simulink model "Assembly1"  (R2019b)
settings: Solver=VariableStepAuto  StartTime=0.0  StopTime=100  FixedStep=0.001
model workspace: external: MATLAB File /home/sydney/Desktop/matlab/simulink/SimpImpCheck/Assembly1_DataFile.m (data not in the file)
undefined symbols (not defined in the file or in its folder): smiData, X, Y, Z
libraries: sm_lib x21, fl_lib x17, nesl_utility x17, ee_lib x3
settings Model: Creator=sydney  LastModifiedBy=sydney

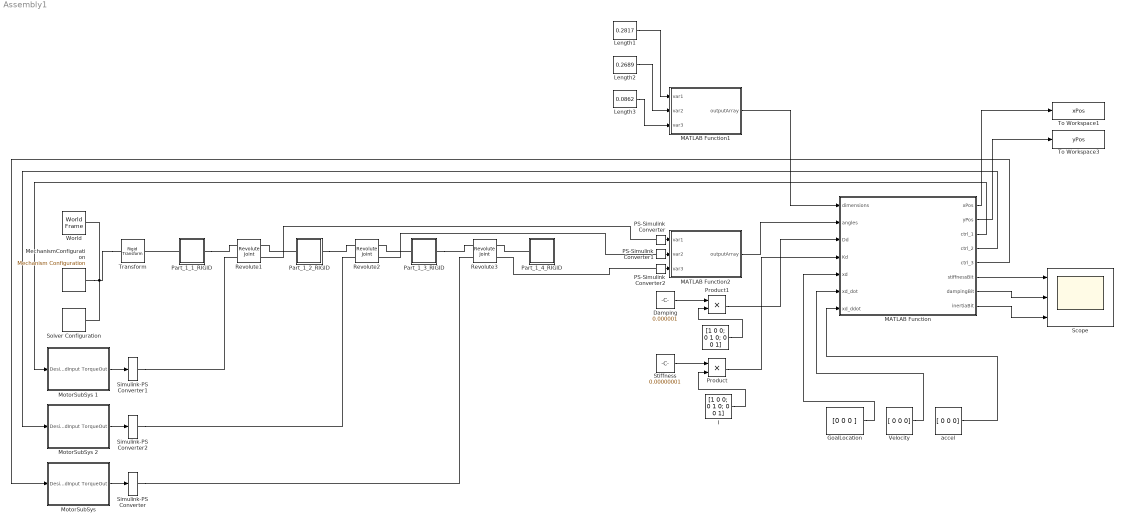
== system Assembly1 ==
  " " : Constant  Value=[1 0 0; 0 1 0; 0 0 1]  VectorParams1D=off
  "Damping " : Constant  Value=0.000001
  GoalLocation : Constant  Value=[0 0 0 ]
  I : Constant  Value=[1 0 0; 0 1 0; 0 0 1]  VectorParams1D=off
  "Length1 " : Constant  Value=0.2817
  "Length2 " : Constant  Value=0.2689
  "Length3 " : Constant  Value=0.0862
  MATLAB Function : MATLAB Function  TreatAsAtomicUnit=on
  MATLAB Function1 : MATLAB Function  TreatAsAtomicUnit=on
  MATLAB Function2 : MATLAB Function  TreatAsAtomicUnit=on
  MechanismConfiguration : sm_lib/Utilities/Mechanism Configuration  UniformGravity=Constant  GravityVector=[0 0 -9.80665]  GravityUnits=m/s^2  LinearizationDelta=0.001
  "MotorSubSys " : Subsystem
  MotorSubSys 1 : Subsystem
  MotorSubSys 2 : Subsystem
  PS-Simulink Converter : nesl_utility/PS-Simulink Converter  PhysicalDomain=network_engine_domain  SubClassName=ps_output  LeftPortType=input  RightPortType=output  PseudoPeriodic=off  Frequencies=[]  Unit=inherit  AffineConversion=off
  PS-Simulink Converter1 : nesl_utility/PS-Simulink Converter  PhysicalDomain=network_engine_domain  SubClassName=ps_output  LeftPortType=input  RightPortType=output  PseudoPeriodic=off  Frequencies=[]  Unit=inherit  AffineConversion=off
  PS-Simulink Converter2 : nesl_utility/PS-Simulink Converter  PhysicalDomain=network_engine_domain  SubClassName=ps_output  LeftPortType=input  RightPortType=output  PseudoPeriodic=off  Frequencies=[]  Unit=inherit  AffineConversion=off
  Part_1_1_RIGID : Subsystem
  Part_1_2_RIGID : Subsystem
  Part_1_3_RIGID : Subsystem
  Part_1_4_RIGID : Subsystem
  Product : Product
  Product1 : Product
  Revolute1 : sm_lib/Joints/Revolute Joint  JointMode=Normal  SenseConstraintForce=off  SenseConstraintForceX=off  SenseConstraintForceY=off  SenseConstraintForceZ=off  SenseConstraintTorque=off  SenseConstraintTorqueX=off  SenseConstraintTorqueY=off  SenseConstraintTorqueZ=off  SenseTotalForce=off  SenseTotalForceX=off  SenseTotalForceY=off  SenseTotalForceZ=off  SenseTotalTorque=off  SenseTotalTorqueX=off  SenseTotalTorqueY=off  SenseTotalTorqueZ=off  CompositeWrenchDir=FollowerOnBase  CompositeWrenchFrame=BaseFrame  EquilibriumPosition=0  EquilibriumPositionUnits=rad  SpringStiffness=0  SpringStiffnessUnits=N*m/rad  DampingCoefficient=0  DampingCoefficientUnits=N*m/(rad/s)  TorqueActuationMode=InputTorque  MotionActuationMode=ComputedMotion  SensePosition=on  SenseVelocity=off  SenseAcceleration=off  SenseTorqueForce=off  SenseLowerLimitTorqueForce=off  SenseUpperLimitTorqueForce=off  LowerLimitSpecify=off  LowerLimitBound=-90  LowerLimitBoundUnits=deg  LowerLimitStiffness=1e4  LowerLimitStiffnessUnits=N*m/deg  LowerLimitDamping=10  LowerLimitDampingUnits=N*m/(deg/s)  LowerLimitTransitionRegionWidth=0.1  LowerLimitTransitionRegionWidthUnits=deg  UpperLimitSpecify=off  UpperLimitBound=90  UpperLimitBoundUnits=deg  UpperLimitStiffness=1e4  UpperLimitStiffnessUnits=N*m/deg  UpperLimitDamping=10  UpperLimitDampingUnits=N*m/(deg/s)  UpperLimitTransitionRegionWidth=0.1  UpperLimitTransitionRegionWidthUnits=deg  PositionTargetSpecify=on  PositionTargetPriority=Low  PositionTargetValue=smiData.RevoluteJoint(2).Rz.Pos  PositionTargetValueUnits=deg  VelocityTargetSpecify=off  VelocityTargetPriority=High  VelocityTargetValue=0  VelocityTargetValueUnits=deg/s
  Revolute2 : sm_lib/Joints/Revolute Joint  JointMode=Normal  SenseConstraintForce=off  SenseConstraintForceX=off  SenseConstraintForceY=off  SenseConstraintForceZ=off  SenseConstraintTorque=off  SenseConstraintTorqueX=off  SenseConstraintTorqueY=off  SenseConstraintTorqueZ=off  SenseTotalForce=off  SenseTotalForceX=off  SenseTotalForceY=off  SenseTotalForceZ=off  SenseTotalTorque=off  SenseTotalTorqueX=off  SenseTotalTorqueY=off  SenseTotalTorqueZ=off  CompositeWrenchDir=FollowerOnBase  CompositeWrenchFrame=BaseFrame  EquilibriumPosition=0  EquilibriumPositionUnits=rad  SpringStiffness=0  SpringStiffnessUnits=N*m/rad  DampingCoefficient=0  DampingCoefficientUnits=N*m/(rad/s)  TorqueActuationMode=InputTorque  MotionActuationMode=ComputedMotion  SensePosition=on  SenseVelocity=off  SenseAcceleration=off  SenseTorqueForce=off  SenseLowerLimitTorqueForce=off  SenseUpperLimitTorqueForce=off  LowerLimitSpecify=off  LowerLimitBound=-90  LowerLimitBoundUnits=deg  LowerLimitStiffness=1e4  LowerLimitStiffnessUnits=N*m/deg  LowerLimitDamping=10  LowerLimitDampingUnits=N*m/(deg/s)  LowerLimitTransitionRegionWidth=0.1  LowerLimitTransitionRegionWidthUnits=deg  UpperLimitSpecify=off  UpperLimitBound=90  UpperLimitBoundUnits=deg  UpperLimitStiffness=1e4  UpperLimitStiffnessUnits=N*m/deg  UpperLimitDamping=10  UpperLimitDampingUnits=N*m/(deg/s)  UpperLimitTransitionRegionWidth=0.1  UpperLimitTransitionRegionWidthUnits=deg  PositionTargetSpecify=on  PositionTargetPriority=Low  PositionTargetValue=smiData.RevoluteJoint(3).Rz.Pos  PositionTargetValueUnits=deg  VelocityTargetSpecify=off  VelocityTargetPriority=High  VelocityTargetValue=0  VelocityTargetValueUnits=deg/s
  Revolute3 : sm_lib/Joints/Revolute Joint  JointMode=Normal  SenseConstraintForce=off  SenseConstraintForceX=off  SenseConstraintForceY=off  SenseConstraintForceZ=off  SenseConstraintTorque=off  SenseConstraintTorqueX=off  SenseConstraintTorqueY=off  SenseConstraintTorqueZ=off  SenseTotalForce=off  SenseTotalForceX=off  SenseTotalForceY=off  SenseTotalForceZ=off  SenseTotalTorque=off  SenseTotalTorqueX=off  SenseTotalTorqueY=off  SenseTotalTorqueZ=off  CompositeWrenchDir=FollowerOnBase  CompositeWrenchFrame=BaseFrame  EquilibriumPosition=0  EquilibriumPositionUnits=rad  SpringStiffness=0  SpringStiffnessUnits=N*m/rad  DampingCoefficient=0  DampingCoefficientUnits=N*m/(rad/s)  TorqueActuationMode=InputTorque  MotionActuationMode=ComputedMotion  SensePosition=on  SenseVelocity=off  SenseAcceleration=off  SenseTorqueForce=off  SenseLowerLimitTorqueForce=off  SenseUpperLimitTorqueForce=off  LowerLimitSpecify=off  LowerLimitBound=-90  LowerLimitBoundUnits=deg  LowerLimitStiffness=1e4  LowerLimitStiffnessUnits=N*m/deg  LowerLimitDamping=10  LowerLimitDampingUnits=N*m/(deg/s)  LowerLimitTransitionRegionWidth=0.1  LowerLimitTransitionRegionWidthUnits=deg  UpperLimitSpecify=off  UpperLimitBound=90  UpperLimitBoundUnits=deg  UpperLimitStiffness=1e4  UpperLimitStiffnessUnits=N*m/deg  UpperLimitDamping=10  UpperLimitDampingUnits=N*m/(deg/s)  UpperLimitTransitionRegionWidth=0.1  UpperLimitTransitionRegionWidthUnits=deg  PositionTargetSpecify=on  PositionTargetPriority=Low  PositionTargetValue=smiData.RevoluteJoint(1).Rz.Pos  PositionTargetValueUnits=deg  VelocityTargetSpecify=off  VelocityTargetPriority=High  VelocityTargetValue=0  VelocityTargetValueUnits=deg/s
  Scope : Scope  NumInputPorts=3
  Simulink-PS Converter : nesl_utility/Simulink-PS Converter  PhysicalDomain=network_engine_domain  SubClassName=ps_input  LeftPortType=input  RightPortType=output  PseudoPeriodic=off  Frequencies=[]  NoiseDistribution=none  NoiseParameters=[]  Unit=N*m  AffineConversion=off  FilteringAndDerivatives=provide  SimscapeFilterOrder=1  InputFilterTimeConstant=0.001  UdotUserProvided=0
  Simulink-PS Converter1 : nesl_utility/Simulink-PS Converter  PhysicalDomain=network_engine_domain  SubClassName=ps_input  LeftPortType=input  RightPortType=output  PseudoPeriodic=off  Frequencies=[]  NoiseDistribution=none  NoiseParameters=[]  Unit=N*m  AffineConversion=off  FilteringAndDerivatives=provide  SimscapeFilterOrder=1  InputFilterTimeConstant=0.001  UdotUserProvided=0
  Simulink-PS Converter2 : nesl_utility/Simulink-PS Converter  PhysicalDomain=network_engine_domain  SubClassName=ps_input  LeftPortType=input  RightPortType=output  PseudoPeriodic=off  Frequencies=[]  NoiseDistribution=none  NoiseParameters=[]  Unit=N*m  AffineConversion=off  FilteringAndDerivatives=provide  SimscapeFilterOrder=1  InputFilterTimeConstant=0.001  UdotUserProvided=0
  Solver Configuration : nesl_utility/Solver Configuration  PhysicalDomain=network_engine_domain  SubClassName=solver  LeftPortType=input  RightPortType=generic  Tones=[]  Harmonics=[]  SimulateNoise=off  Profile=off  UseLocalSampling=off  EnableSwitchedLinearOptims=on  FrequencyDomain=off  UseCCode=off  RelTol=0.001  AbsTol=1e-06  MinStep=1e-09  ToWorkspace=off  RevertToSquareIcSolve=off  NumHomotopyIterations=100  PhasorMode=off  PhasorModeNumHarmonics=1  DoDC=off  ResidualTolerance=1e-09  UseLocalSolver=off  LocalSolverChoice=NE_BACKWARD_EULER_ADVANCER  LocalSolverSampleTime=0.001  DoFixedCost=off  MaxNonlinIter=3  MaxModeIter=2  LinearAlgebra=auto  EquationFormulation=NE_TIME_EF  DelaysMemoryBudget=1024  AutomaticFiltering=on  FilteringTimeConstant=0.001  PartitionStorageMethod=AS_NEEDED  PartitionMemoryBudget=1024  PartitionMethod=ROBUST
  "Stiffness " : Constant  Value=0.00000001
  To Workspace1 : ToWorkspace  VariableName=xPos  SaveFormat=Structure With Time  SampleTime=-1
  To Workspace3 : ToWorkspace  VariableName=yPos  SaveFormat=Structure With Time  SampleTime=-1
  Transform : sm_lib/Frames and Transforms/Rigid Transform  TranslationMethod=Cartesian  TranslationStandardOffset=0  TranslationLengthUnit=mm  TranslationStandardAxis=+Z  TranslationCartesianOffset=smiData.RigidTransform(2).translation  TranslationROffset=0  TranslationROffsetUnits=m  TranslationZOffset=0  TranslationZOffsetUnits=m  TranslationThetaOffset=0  TranslationThetaOffsetUnits=deg  RotationMethod=ArbitraryAxis  RotationAngleUnits=rad  RotationStandardAxis=+Z  RotationAngle=smiData.RigidTransform(2).angle  RotationArbitraryAxis=smiData.RigidTransform(2).axis  FollAlignAxisA=+X  BaseAlignAxisA=+Y  FollAlignAxisB=+Y  BaseAlignAxisB=+Z  RotationSequenceAxes=FollowerAxes  RotationSequence=XYX  RotationSequenceAngles=[0 0 0]  RotationSequenceAnglesUnits=deg  RotationMatrix=[1 0 0; 0 1 0; 0 0 1]
  "Velocity " : Constant  Value=[ 0 0 0]
  World : sm_lib/Frames and Transforms/World Frame
  "accel " : Constant  Value=[ 0 0 0]
  wires:
  I/1 -> Product/2
  MATLAB Function/3(ctrl_1) -> MotorSubSys 1/1("DesiredInput ")
  "MotorSubSys "/1("TorqueOut ") -> Simulink-PS Converter/1
  MotorSubSys 2/1("TorqueOut ") -> Simulink-PS Converter2/1
  "Length2 "/1 -> MATLAB Function1/2(var2)
  MATLAB Function/4(ctrl_2) -> MotorSubSys 2/1("DesiredInput ")
  MotorSubSys 1/1("TorqueOut ") -> Simulink-PS Converter1/1
  MATLAB Function2/1(outputArray) -> MATLAB Function/2(angles)
  "Length3 "/1 -> MATLAB Function1/3(var3)
  PS-Simulink Converter2/1 -> MATLAB Function2/3(var3)
  GoalLocation/1 -> MATLAB Function/5(xd)
  Product1/1 -> MATLAB Function/3(Dd)
  "Velocity "/1 -> MATLAB Function/6(xd_dot)
  MATLAB Function/5(ctrl_3) -> "MotorSubSys "/1("DesiredInput ")
  PS-Simulink Converter/1 -> MATLAB Function2/1(var1)
  PS-Simulink Converter1/1 -> MATLAB Function2/2(var2)
  MATLAB Function/1(xPos) -> To Workspace1/1
  MATLAB Function1/1(outputArray) -> MATLAB Function/1(dimensions)
  Product/1 -> MATLAB Function/4(Kd)
  "Stiffness "/1 -> Product/1
  "Damping "/1 -> Product1/1
  MATLAB Function/2(yPos) -> To Workspace3/1
  " "/1 -> Product1/2
  "Length1 "/1 -> MATLAB Function1/1(var1)
  "accel "/1 -> MATLAB Function/7(xd_ddot)
  MATLAB Function/6(stiffnessBit) -> Scope/1
  MATLAB Function/7(dampingBit) -> Scope/2
  MATLAB Function/8(inertiaBit) -> Scope/3
  connections:
  Transform/LConn1 -- MechanismConfiguration/RConn1 -- Solver Configuration/RConn1 -- World/RConn1
  Part_1_1_RIGID/LConn1 -- Transform/RConn1
  Part_1_3_RIGID/RConn1 -- Revolute3/LConn1
  Part_1_4_RIGID/LConn1 -- Revolute3/RConn1
  Part_1_1_RIGID/RConn1 -- Revolute1/LConn1
  Part_1_2_RIGID/LConn1 -- Revolute1/RConn1
  Part_1_2_RIGID/RConn1 -- Revolute2/LConn1
  Part_1_3_RIGID/LConn1 -- Revolute2/RConn1
  Simulink-PS Converter1/RConn1 -- Revolute1/LConn2
  Simulink-PS Converter2/RConn1 -- Revolute2/LConn2
  Simulink-PS Converter/RConn1 -- Revolute3/LConn2
  PS-Simulink Converter/LConn1 -- Revolute1/RConn2
  PS-Simulink Converter1/LConn1 -- Revolute2/RConn2
  PS-Simulink Converter2/LConn1 -- Revolute3/RConn2

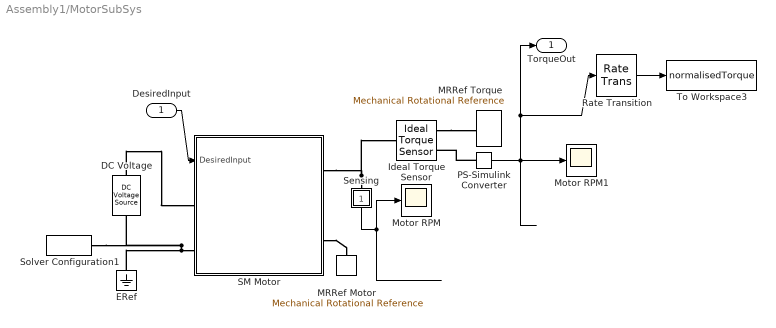
== system Assembly1/MotorSubSys  ==
  "DesiredInput " : Inport
  DC Voltage : fl_lib/Electrical/Electrical Sources/DC Voltage Source  v0=48 V
  ERef : fl_lib/Electrical/Electrical Elements/Electrical Reference
  Ideal Torque Sensor : fl_lib/Mechanical/Mechanical Sensors/Ideal Torque Sensor
  MRRef Motor : fl_lib/Mechanical/Rotational Elements/Mechanical Rotational Reference
  MRRef Torque : fl_lib/Mechanical/Rotational Elements/Mechanical Rotational Reference
  Motor RPM : Scope
  Motor RPM1 : Scope
  PS-Simulink Converter : nesl_utility/PS-Simulink Converter  PhysicalDomain=network_engine_domain  SubClassName=ps_output  LeftPortType=input  RightPortType=output  PseudoPeriodic=off  Frequencies=[]  Unit=inherit  AffineConversion=off
  Rate Transition : RateTransition  OutPortSampleTime=1e-3
  SM Motor : Subsystem  Tag=PublishSubsystem
      mask Display:
      | % Circle, in/out, and 'M'
      | image(imread('ssc_dcmotor_maskicon.png'));
      | 
      | % % Circle
      | % plot(sin(0:0.1:2.2*pi)*0.9,cos(0:0.1:2.2*pi)*0.9);
      | %
      | % % In/out
      | % plot([-1.3 -0.9],[0 0]);
      | % plot([1.3 0.9],[0 0]);
      | %
      | % % 'M'
      | % plot([0.5 0.5],[-0.5 0.5]);
      | % plot([-0.5 -0.5],[-0.5 0.5]);
      | % plot([0.5 0],[0.5 -0.5]);
      | % plot([-0.5 0],[0.5 -0.5]);
      | 
      | % Plot points to set plot range
      | color('white');plot(1.5,1.5);plot(-1.5,-1.5)
      | color('black');
      | 
      | port_label('RConn',1,'R');
      | port_label('RConn',2,'C');
      | port_label('LConn',1,'V+');
      | port_label('LConn',2,'V-');
  Sensing : Subsystem
      mask Display: disp('w');
  Solver Configuration1 : nesl_utility/Solver Configuration  PhysicalDomain=network_engine_domain  SubClassName=solver  LeftPortType=input  RightPortType=generic  Tones=[]  Harmonics=[]  SimulateNoise=off  Profile=off  UseLocalSampling=off  EnableSwitchedLinearOptims=on  FrequencyDomain=off  UseCCode=off  RelTol=0.001  AbsTol=1e-06  MinStep=1e-09  ToWorkspace=off  RevertToSquareIcSolve=off  NumHomotopyIterations=100  PhasorMode=off  PhasorModeNumHarmonics=1  DoDC=off  ResidualTolerance=1e-9  UseLocalSolver=off  LocalSolverChoice=NE_BACKWARD_EULER_ADVANCER  LocalSolverSampleTime=.001  DoFixedCost=off  MaxNonlinIter=3  MaxModeIter=2  LinearAlgebra=auto  EquationFormulation=NE_TIME_EF  DelaysMemoryBudget=1024  AutomaticFiltering=on  FilteringTimeConstant=0.001  PartitionStorageMethod=AS_NEEDED  PartitionMemoryBudget=1024  PartitionMethod=FAST
  To Workspace3 : ToWorkspace  VariableName=normalisedTorque  SaveFormat=Structure With Time  SampleTime=-1
  "TorqueOut " : Outport
  wires:
  Sensing/1("rotation sensor ") -> Motor RPM/1
  Rate Transition/1 -> To Workspace3/1
  PS-Simulink Converter/1 -> "TorqueOut "/1, Rate Transition/1, Motor RPM1/1
  "DesiredInput "/1 -> SM Motor/1("DesiredInput ")
  connections:
  PS-Simulink Converter/LConn1 -- Ideal Torque Sensor/RConn2
  SM Motor/LConn2 -- DC Voltage/RConn1 -- Solver Configuration1/RConn1 -- ERef/LConn1
  DC Voltage/LConn1 -- SM Motor/LConn1
  Sensing/LConn1 -- Ideal Torque Sensor/LConn1 -- SM Motor/RConn1
  SM Motor/RConn2 -- MRRef Motor/LConn1
  Ideal Torque Sensor/RConn1 -- MRRef Torque/LConn1

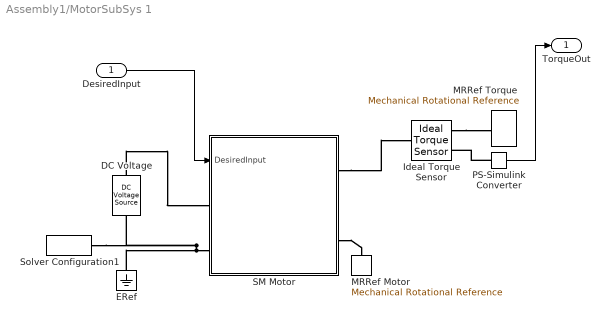
== system Assembly1/MotorSubSys 1 ==
  "DesiredInput " : Inport
  DC Voltage : fl_lib/Electrical/Electrical Sources/DC Voltage Source  v0=48 V
  ERef : fl_lib/Electrical/Electrical Elements/Electrical Reference
  Ideal Torque Sensor : fl_lib/Mechanical/Mechanical Sensors/Ideal Torque Sensor
  MRRef Motor : fl_lib/Mechanical/Rotational Elements/Mechanical Rotational Reference
  MRRef Torque : fl_lib/Mechanical/Rotational Elements/Mechanical Rotational Reference
  PS-Simulink Converter : nesl_utility/PS-Simulink Converter  PhysicalDomain=network_engine_domain  SubClassName=ps_output  LeftPortType=input  RightPortType=output  PseudoPeriodic=off  Frequencies=[]  Unit=inherit  AffineConversion=off
  SM Motor : Subsystem  Tag=PublishSubsystem
      mask Display:
      | % Circle, in/out, and 'M'
      | image(imread('ssc_dcmotor_maskicon.png'));
      | 
      | % % Circle
      | % plot(sin(0:0.1:2.2*pi)*0.9,cos(0:0.1:2.2*pi)*0.9);
      | %
      | % % In/out
      | % plot([-1.3 -0.9],[0 0]);
      | % plot([1.3 0.9],[0 0]);
      | %
      | % % 'M'
      | % plot([0.5 0.5],[-0.5 0.5]);
      | % plot([-0.5 -0.5],[-0.5 0.5]);
      | % plot([0.5 0],[0.5 -0.5]);
      | % plot([-0.5 0],[0.5 -0.5]);
      | 
      | % Plot points to set plot range
      | color('white');plot(1.5,1.5);plot(-1.5,-1.5)
      | color('black');
      | 
      | port_label('RConn',1,'R');
      | port_label('RConn',2,'C');
      | port_label('LConn',1,'V+');
      | port_label('LConn',2,'V-');
  Solver Configuration1 : nesl_utility/Solver Configuration  PhysicalDomain=network_engine_domain  SubClassName=solver  LeftPortType=input  RightPortType=generic  Tones=[]  Harmonics=[]  SimulateNoise=off  Profile=off  UseLocalSampling=off  EnableSwitchedLinearOptims=on  FrequencyDomain=off  UseCCode=off  RelTol=0.001  AbsTol=1e-06  MinStep=1e-09  ToWorkspace=off  RevertToSquareIcSolve=off  NumHomotopyIterations=100  PhasorMode=off  PhasorModeNumHarmonics=1  DoDC=off  ResidualTolerance=1e-9  UseLocalSolver=off  LocalSolverChoice=NE_BACKWARD_EULER_ADVANCER  LocalSolverSampleTime=.001  DoFixedCost=off  MaxNonlinIter=3  MaxModeIter=2  LinearAlgebra=auto  EquationFormulation=NE_TIME_EF  DelaysMemoryBudget=1024  AutomaticFiltering=on  FilteringTimeConstant=0.001  PartitionStorageMethod=AS_NEEDED  PartitionMemoryBudget=1024  PartitionMethod=FAST
  "TorqueOut " : Outport
  wires:
  PS-Simulink Converter/1 -> "TorqueOut "/1
  "DesiredInput "/1 -> SM Motor/1("DesiredInput ")
  connections:
  PS-Simulink Converter/LConn1 -- Ideal Torque Sensor/RConn2
  SM Motor/LConn2 -- DC Voltage/RConn1 -- Solver Configuration1/RConn1 -- ERef/LConn1
  DC Voltage/LConn1 -- SM Motor/LConn1
  SM Motor/RConn1 -- Ideal Torque Sensor/LConn1
  SM Motor/RConn2 -- MRRef Motor/LConn1
  Ideal Torque Sensor/RConn1 -- MRRef Torque/LConn1

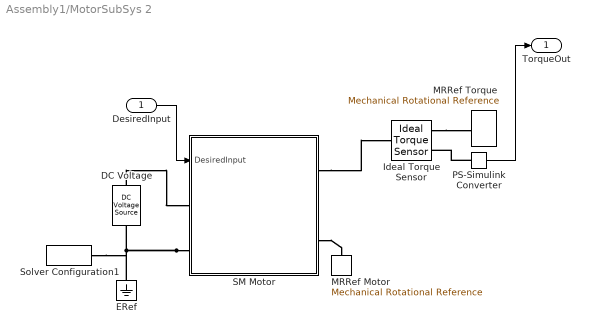
== system Assembly1/MotorSubSys 2 ==
  "DesiredInput " : Inport
  DC Voltage : fl_lib/Electrical/Electrical Sources/DC Voltage Source  v0=48 V
  ERef : fl_lib/Electrical/Electrical Elements/Electrical Reference
  Ideal Torque Sensor : fl_lib/Mechanical/Mechanical Sensors/Ideal Torque Sensor
  MRRef Motor : fl_lib/Mechanical/Rotational Elements/Mechanical Rotational Reference
  MRRef Torque : fl_lib/Mechanical/Rotational Elements/Mechanical Rotational Reference
  PS-Simulink Converter : nesl_utility/PS-Simulink Converter  PhysicalDomain=network_engine_domain  SubClassName=ps_output  LeftPortType=input  RightPortType=output  PseudoPeriodic=off  Frequencies=[]  Unit=inherit  AffineConversion=off
  SM Motor : Subsystem  Tag=PublishSubsystem
      mask Display:
      | % Circle, in/out, and 'M'
      | image(imread('ssc_dcmotor_maskicon.png'));
      | 
      | % % Circle
      | % plot(sin(0:0.1:2.2*pi)*0.9,cos(0:0.1:2.2*pi)*0.9);
      | %
      | % % In/out
      | % plot([-1.3 -0.9],[0 0]);
      | % plot([1.3 0.9],[0 0]);
      | %
      | % % 'M'
      | % plot([0.5 0.5],[-0.5 0.5]);
      | % plot([-0.5 -0.5],[-0.5 0.5]);
      | % plot([0.5 0],[0.5 -0.5]);
      | % plot([-0.5 0],[0.5 -0.5]);
      | 
      | % Plot points to set plot range
      | color('white');plot(1.5,1.5);plot(-1.5,-1.5)
      | color('black');
      | 
      | port_label('RConn',1,'R');
      | port_label('RConn',2,'C');
      | port_label('LConn',1,'V+');
      | port_label('LConn',2,'V-');
  Solver Configuration1 : nesl_utility/Solver Configuration  PhysicalDomain=network_engine_domain  SubClassName=solver  LeftPortType=input  RightPortType=generic  Tones=[]  Harmonics=[]  SimulateNoise=off  Profile=off  UseLocalSampling=off  EnableSwitchedLinearOptims=on  FrequencyDomain=off  UseCCode=off  RelTol=0.001  AbsTol=1e-06  MinStep=1e-09  ToWorkspace=off  RevertToSquareIcSolve=off  NumHomotopyIterations=100  PhasorMode=off  PhasorModeNumHarmonics=1  DoDC=off  ResidualTolerance=1e-9  UseLocalSolver=off  LocalSolverChoice=NE_BACKWARD_EULER_ADVANCER  LocalSolverSampleTime=.001  DoFixedCost=off  MaxNonlinIter=3  MaxModeIter=2  LinearAlgebra=auto  EquationFormulation=NE_TIME_EF  DelaysMemoryBudget=1024  AutomaticFiltering=on  FilteringTimeConstant=0.001  PartitionStorageMethod=AS_NEEDED  PartitionMemoryBudget=1024  PartitionMethod=FAST
  "TorqueOut " : Outport
  wires:
  PS-Simulink Converter/1 -> "TorqueOut "/1
  "DesiredInput "/1 -> SM Motor/1("DesiredInput ")
  connections:
  PS-Simulink Converter/LConn1 -- Ideal Torque Sensor/RConn2
  SM Motor/LConn2 -- DC Voltage/RConn1 -- ERef/LConn1 -- Solver Configuration1/RConn1
  DC Voltage/LConn1 -- SM Motor/LConn1
  SM Motor/RConn1 -- Ideal Torque Sensor/LConn1
  SM Motor/RConn2 -- MRRef Motor/LConn1
  Ideal Torque Sensor/RConn1 -- MRRef Torque/LConn1

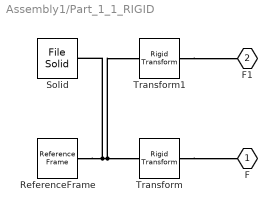
== system Assembly1/Part_1_1_RIGID ==
  ReferenceFrame : sm_lib/Frames and Transforms/Reference Frame
  Solid : sm_lib/Body Elements/File Solid  ExtGeomFileName=Part 11.step  UnitType=FromFile  ExtGeomFileUnits=m  StepReaderType=HEX  ExportEntireGeometry=off  InertiaType=Custom  Mass=smiData.Solid(4).mass  MassUnits=kg  CenterOfMass=smiData.Solid(4).CoM  CenterOfMassUnits=mm  MomentsOfInertia=smiData.Solid(4).MoI  MomentsOfInertiaUnits=kg*mm^2  ProductsOfInertia=smiData.Solid(4).PoI  ProductsOfInertiaUnits=kg*mm^2  BasedOnType=DensityFromFile  Density=1000  DensityUnits=kg/m^3  DoExposeReferenceFrame=on  SerializedFrames=<Frames/>  GraphicType=FromGeometry  MarkerShape=Sphere  MarkerSize=10  GraphicVisPropType=SimpleVisualProperties  GraphicDiffuseColor=smiData.Solid(4).color  GraphicSpecularColor=[0.5 0.5 0.5 1.0]  GraphicAmbientColor=[0.15 0.15 0.15 1.0]  GraphicEmissiveColor=[0.0 0.0 0.0 1.0]  GraphicShininess=75  GraphicOpacity=smiData.Solid(4).opacity
  Transform : sm_lib/Frames and Transforms/Rigid Transform  TranslationMethod=Cartesian  TranslationStandardOffset=0  TranslationLengthUnit=mm  TranslationStandardAxis=+Z  TranslationCartesianOffset=smiData.RigidTransform(1).translation  TranslationROffset=0  TranslationROffsetUnits=m  TranslationZOffset=0  TranslationZOffsetUnits=m  TranslationThetaOffset=0  TranslationThetaOffsetUnits=deg  RotationMethod=ArbitraryAxis  RotationAngleUnits=rad  RotationStandardAxis=+Z  RotationAngle=smiData.RigidTransform(1).angle  RotationArbitraryAxis=smiData.RigidTransform(1).axis  FollAlignAxisA=+X  BaseAlignAxisA=+Y  FollAlignAxisB=+Y  BaseAlignAxisB=+Z  RotationSequenceAxes=FollowerAxes  RotationSequence=XYX  RotationSequenceAngles=[0 0 0]  RotationSequenceAnglesUnits=deg  RotationMatrix=[1 0 0; 0 1 0; 0 0 1]
  Transform1 : sm_lib/Frames and Transforms/Rigid Transform  TranslationMethod=Cartesian  TranslationStandardOffset=0  TranslationLengthUnit=mm  TranslationStandardAxis=+Z  TranslationCartesianOffset=smiData.RigidTransform(5).translation  TranslationROffset=0  TranslationROffsetUnits=m  TranslationZOffset=0  TranslationZOffsetUnits=m  TranslationThetaOffset=0  TranslationThetaOffsetUnits=deg  RotationMethod=ArbitraryAxis  RotationAngleUnits=rad  RotationStandardAxis=+Z  RotationAngle=smiData.RigidTransform(5).angle  RotationArbitraryAxis=smiData.RigidTransform(5).axis  FollAlignAxisA=+X  BaseAlignAxisA=+Y  FollAlignAxisB=+Y  BaseAlignAxisB=+Z  RotationSequenceAxes=FollowerAxes  RotationSequence=XYX  RotationSequenceAngles=[0 0 0]  RotationSequenceAnglesUnits=deg  RotationMatrix=[1 0 0; 0 1 0; 0 0 1]
  F : PMIOPort  Side=Left
  F1 : PMIOPort  Port=2  Side=Right
  connections:
  Solid/RConn1 -- ReferenceFrame/RConn1 -- Transform/LConn1 -- Transform1/LConn1
  Transform/RConn1 -- F/RConn1
  Transform1/RConn1 -- F1/RConn1

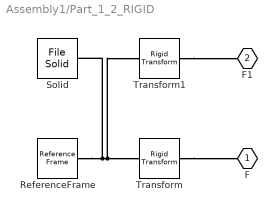
== system Assembly1/Part_1_2_RIGID ==
  ReferenceFrame : sm_lib/Frames and Transforms/Reference Frame
  Solid : sm_lib/Body Elements/File Solid  ExtGeomFileName=Part 13.step  UnitType=FromFile  ExtGeomFileUnits=m  StepReaderType=HEX  ExportEntireGeometry=off  InertiaType=Custom  Mass=smiData.Solid(1).mass  MassUnits=kg  CenterOfMass=smiData.Solid(1).CoM  CenterOfMassUnits=mm  MomentsOfInertia=smiData.Solid(1).MoI  MomentsOfInertiaUnits=kg*mm^2  ProductsOfInertia=smiData.Solid(1).PoI  ProductsOfInertiaUnits=kg*mm^2  BasedOnType=DensityFromFile  Density=1000  DensityUnits=kg/m^3  DoExposeReferenceFrame=on  SerializedFrames=<Frames/>  GraphicType=FromGeometry  MarkerShape=Sphere  MarkerSize=10  GraphicVisPropType=SimpleVisualProperties  GraphicDiffuseColor=smiData.Solid(1).color  GraphicSpecularColor=[0.5 0.5 0.5 1.0]  GraphicAmbientColor=[0.15 0.15 0.15 1.0]  GraphicEmissiveColor=[0.0 0.0 0.0 1.0]  GraphicShininess=75  GraphicOpacity=smiData.Solid(1).opacity
  Transform : sm_lib/Frames and Transforms/Rigid Transform  TranslationMethod=Cartesian  TranslationStandardOffset=0  TranslationLengthUnit=mm  TranslationStandardAxis=+Z  TranslationCartesianOffset=smiData.RigidTransform(6).translation  TranslationROffset=0  TranslationROffsetUnits=m  TranslationZOffset=0  TranslationZOffsetUnits=m  TranslationThetaOffset=0  TranslationThetaOffsetUnits=deg  RotationMethod=ArbitraryAxis  RotationAngleUnits=rad  RotationStandardAxis=+Z  RotationAngle=smiData.RigidTransform(6).angle  RotationArbitraryAxis=smiData.RigidTransform(6).axis  FollAlignAxisA=+X  BaseAlignAxisA=+Y  FollAlignAxisB=+Y  BaseAlignAxisB=+Z  RotationSequenceAxes=FollowerAxes  RotationSequence=XYX  RotationSequenceAngles=[0 0 0]  RotationSequenceAnglesUnits=deg  RotationMatrix=[1 0 0; 0 1 0; 0 0 1]
  Transform1 : sm_lib/Frames and Transforms/Rigid Transform  TranslationMethod=Cartesian  TranslationStandardOffset=0  TranslationLengthUnit=mm  TranslationStandardAxis=+Z  TranslationCartesianOffset=smiData.RigidTransform(7).translation  TranslationROffset=0  TranslationROffsetUnits=m  TranslationZOffset=0  TranslationZOffsetUnits=m  TranslationThetaOffset=0  TranslationThetaOffsetUnits=deg  RotationMethod=ArbitraryAxis  RotationAngleUnits=rad  RotationStandardAxis=+Z  RotationAngle=smiData.RigidTransform(7).angle  RotationArbitraryAxis=smiData.RigidTransform(7).axis  FollAlignAxisA=+X  BaseAlignAxisA=+Y  FollAlignAxisB=+Y  BaseAlignAxisB=+Z  RotationSequenceAxes=FollowerAxes  RotationSequence=XYX  RotationSequenceAngles=[0 0 0]  RotationSequenceAnglesUnits=deg  RotationMatrix=[1 0 0; 0 1 0; 0 0 1]
  F : PMIOPort  Side=Left
  F1 : PMIOPort  Port=2  Side=Right
  connections:
  Solid/RConn1 -- ReferenceFrame/RConn1 -- Transform/LConn1 -- Transform1/LConn1
  Transform/RConn1 -- F/RConn1
  Transform1/RConn1 -- F1/RConn1

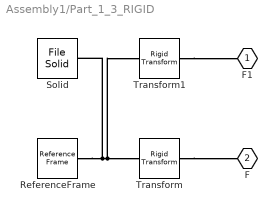
== system Assembly1/Part_1_3_RIGID ==
  ReferenceFrame : sm_lib/Frames and Transforms/Reference Frame
  Solid : sm_lib/Body Elements/File Solid  ExtGeomFileName=Part 12.step  UnitType=FromFile  ExtGeomFileUnits=m  StepReaderType=HEX  ExportEntireGeometry=off  InertiaType=Custom  Mass=smiData.Solid(3).mass  MassUnits=kg  CenterOfMass=smiData.Solid(3).CoM  CenterOfMassUnits=mm  MomentsOfInertia=smiData.Solid(3).MoI  MomentsOfInertiaUnits=kg*mm^2  ProductsOfInertia=smiData.Solid(3).PoI  ProductsOfInertiaUnits=kg*mm^2  BasedOnType=DensityFromFile  Density=1000  DensityUnits=kg/m^3  DoExposeReferenceFrame=on  SerializedFrames=<Frames/>  GraphicType=FromGeometry  MarkerShape=Sphere  MarkerSize=10  GraphicVisPropType=SimpleVisualProperties  GraphicDiffuseColor=smiData.Solid(3).color  GraphicSpecularColor=[0.5 0.5 0.5 1.0]  GraphicAmbientColor=[0.15 0.15 0.15 1.0]  GraphicEmissiveColor=[0.0 0.0 0.0 1.0]  GraphicShininess=75  GraphicOpacity=smiData.Solid(3).opacity
  Transform : sm_lib/Frames and Transforms/Rigid Transform  TranslationMethod=Cartesian  TranslationStandardOffset=0  TranslationLengthUnit=mm  TranslationStandardAxis=+Z  TranslationCartesianOffset=smiData.RigidTransform(3).translation  TranslationROffset=0  TranslationROffsetUnits=m  TranslationZOffset=0  TranslationZOffsetUnits=m  TranslationThetaOffset=0  TranslationThetaOffsetUnits=deg  RotationMethod=ArbitraryAxis  RotationAngleUnits=rad  RotationStandardAxis=+Z  RotationAngle=smiData.RigidTransform(3).angle  RotationArbitraryAxis=smiData.RigidTransform(3).axis  FollAlignAxisA=+X  BaseAlignAxisA=+Y  FollAlignAxisB=+Y  BaseAlignAxisB=+Z  RotationSequenceAxes=FollowerAxes  RotationSequence=XYX  RotationSequenceAngles=[0 0 0]  RotationSequenceAnglesUnits=deg  RotationMatrix=[1 0 0; 0 1 0; 0 0 1]
  Transform1 : sm_lib/Frames and Transforms/Rigid Transform  TranslationMethod=Cartesian  TranslationStandardOffset=0  TranslationLengthUnit=mm  TranslationStandardAxis=+Z  TranslationCartesianOffset=smiData.RigidTransform(8).translation  TranslationROffset=0  TranslationROffsetUnits=m  TranslationZOffset=0  TranslationZOffsetUnits=m  TranslationThetaOffset=0  TranslationThetaOffsetUnits=deg  RotationMethod=ArbitraryAxis  RotationAngleUnits=rad  RotationStandardAxis=+Z  RotationAngle=smiData.RigidTransform(8).angle  RotationArbitraryAxis=smiData.RigidTransform(8).axis  FollAlignAxisA=+X  BaseAlignAxisA=+Y  FollAlignAxisB=+Y  BaseAlignAxisB=+Z  RotationSequenceAxes=FollowerAxes  RotationSequence=XYX  RotationSequenceAngles=[0 0 0]  RotationSequenceAnglesUnits=deg  RotationMatrix=[1 0 0; 0 1 0; 0 0 1]
  F1 : PMIOPort  Side=Left
  F : PMIOPort  Port=2  Side=Right
  connections:
  Solid/RConn1 -- ReferenceFrame/RConn1 -- Transform/LConn1 -- Transform1/LConn1
  Transform/RConn1 -- F/RConn1
  Transform1/RConn1 -- F1/RConn1

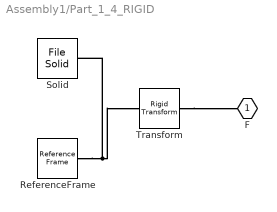
== system Assembly1/Part_1_4_RIGID ==
  ReferenceFrame : sm_lib/Frames and Transforms/Reference Frame
  Solid : sm_lib/Body Elements/File Solid  ExtGeomFileName=Part 1.step  UnitType=FromFile  ExtGeomFileUnits=m  StepReaderType=HEX  ExportEntireGeometry=off  InertiaType=Custom  Mass=smiData.Solid(2).mass  MassUnits=kg  CenterOfMass=smiData.Solid(2).CoM  CenterOfMassUnits=mm  MomentsOfInertia=smiData.Solid(2).MoI  MomentsOfInertiaUnits=kg*mm^2  ProductsOfInertia=smiData.Solid(2).PoI  ProductsOfInertiaUnits=kg*mm^2  BasedOnType=DensityFromFile  Density=1000  DensityUnits=kg/m^3  DoExposeReferenceFrame=on  SerializedFrames=<Frames/>  GraphicType=FromGeometry  MarkerShape=Sphere  MarkerSize=10  GraphicVisPropType=SimpleVisualProperties  GraphicDiffuseColor=smiData.Solid(2).color  GraphicSpecularColor=[0.5 0.5 0.5 1.0]  GraphicAmbientColor=[0.15 0.15 0.15 1.0]  GraphicEmissiveColor=[0.0 0.0 0.0 1.0]  GraphicShininess=75  GraphicOpacity=smiData.Solid(2).opacity
  Transform : sm_lib/Frames and Transforms/Rigid Transform  TranslationMethod=Cartesian  TranslationStandardOffset=0  TranslationLengthUnit=mm  TranslationStandardAxis=+Z  TranslationCartesianOffset=smiData.RigidTransform(4).translation  TranslationROffset=0  TranslationROffsetUnits=m  TranslationZOffset=0  TranslationZOffsetUnits=m  TranslationThetaOffset=0  TranslationThetaOffsetUnits=deg  RotationMethod=ArbitraryAxis  RotationAngleUnits=rad  RotationStandardAxis=+Z  RotationAngle=smiData.RigidTransform(4).angle  RotationArbitraryAxis=smiData.RigidTransform(4).axis  FollAlignAxisA=+X  BaseAlignAxisA=+Y  FollAlignAxisB=+Y  BaseAlignAxisB=+Z  RotationSequenceAxes=FollowerAxes  RotationSequence=XYX  RotationSequenceAngles=[0 0 0]  RotationSequenceAnglesUnits=deg  RotationMatrix=[1 0 0; 0 1 0; 0 0 1]
  F : PMIOPort  Side=Left
  connections:
  Solid/RConn1 -- ReferenceFrame/RConn1 -- Transform/LConn1
  Transform/RConn1 -- F/RConn1

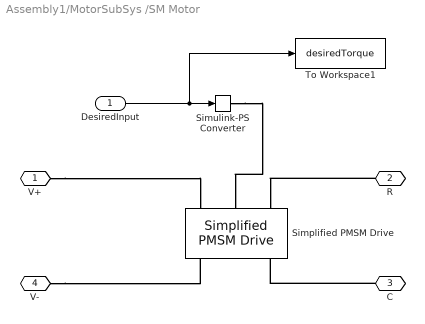
== system Assembly1/MotorSubSys /SM Motor ==
  "DesiredInput " : Inport
  Simplified PMSM Drive : ee_lib/Electromechanical/Permanent Magnet/Simplified PMSM Drive  torque_speed_param=2  w_t=[0, 3750, 7500, 8000] rpm  T_t=[.09, .08, .07, 0] N*m  torque_max=1490 mN*m  power_max=285.6 W  Tc=7.99 ms  losses_param=1  eff=86.5  w_eff=1960 rpm  T_eff=65.373 mN*m  Piron=1.8338 W  Pbase=0 W  w_eff_vec=[-8000, -4000, 0, 4000, 8000] rpm  T_eff_vec=[0, .03, .06, .09] N*m  v_eff_vec=[100, 250, 400] V  losses_mat=[1.49, 1.67, 2.21, 3.1; .42, .69, 1.14, 2.03; .06, .24, .78, 1.68; .42, .69, 1.14, 2.03; 1.49, 1.67, 2.21, 3.1] W  efficiency_mat=[95, 95, 95, 95; 95, 95, 95, 95; 95, 95, 95, 95; 95, 95, 95, 95; 95, 95, 95, 95]  losses_mat_3D=ones(5, 4, 3) W  efficiency_mat_3D=95 * ones(5, 4, 3)  Res=0 Ohm  J=5100 g*cm^2  lam=1e-5 N*m/(rad/s)  speed0=0 rpm  faulted_specify=off  faulted_priority=None  faulted=0  faulted_nominal_specify=off  faulted_nominal_unit=1  faulted_nominal_value=1  alpha=3.93e-3 1/K  Tmeas=25 degC  Tmeas2=125 degC  losses_mat_T2=[1.49, 1.74, 2.49, 3.74; .42, .67, 1.42, 2.67; .06, .31, 1.06, 2.31; .42, .67, 1.42, 2.67; 1.49, 1.74, 2.49, 3.74] W  efficiency_mat_T2=[95, 95, 95, 95; 95, 95, 95, 95; 95, 95, 95, 95; 95, 95, 95, 95; 95, 95, 95, 95]  losses_mat_3D_T2=ones(5, 4, 3) W  efficiency_mat_3D_T2=95 * ones(5, 4, 3)  thermal_mass=100 J/K  initial_temperature=25 degC  fault_condition=1  fault_threshold=0.5
      settings: SourceProductName=Simscape Electrical  SourceProductBaseCode=PS  InternalSimscapePortConfiguration="{\"Bottom\":[],\"Left\":[{\"id\":\"Vp\",\"label\":\"+\",\"type\":\"foundation.electrical.electrical\"},{\"id\":\"Tr\",\"label\":\"Tr\",\"type\":\"input\"},{\"id\":\"R\",\"label\":\"R\",\"type\":\"foundation.mechanical.rotational.rotational\"}],\"Right\":[{\"id\":\"Vm\",\"label\":\"-\",\"type\":\"foundation.electrical.electrical\"},{\"id\":\"Omega\",\"label\":\"w\",\"type\":\"output\"},{\"id\":\"C\",\"label\":\"C\",\"type\":\"foundation.mechanical.rotational.rotational\"}],\"Top\":[]}"
  Simulink-PS Converter : nesl_utility/Simulink-PS Converter  PhysicalDomain=network_engine_domain  SubClassName=ps_input  LeftPortType=input  RightPortType=output  PseudoPeriodic=off  Frequencies=[]  NoiseDistribution=none  NoiseParameters=[]  Unit=1  AffineConversion=off  FilteringAndDerivatives=provide  SimscapeFilterOrder=1  InputFilterTimeConstant=0.001  UdotUserProvided=0
  To Workspace1 : ToWorkspace  VariableName=desiredTorque  SampleTime=-1
  V+ : PMIOPort  Side=Left
  R : PMIOPort  Port=2  Side=Right
  C : PMIOPort  Port=3  Side=Right
  V- : PMIOPort  Port=4  Side=Left
  wires:
  "DesiredInput "/1 -> To Workspace1/1, Simulink-PS Converter/1
  connections:
  V-/RConn1 -- Simplified PMSM Drive/RConn1
  V+/RConn1 -- Simplified PMSM Drive/LConn1
  R/RConn1 -- Simplified PMSM Drive/LConn3
  Simulink-PS Converter/RConn1 -- Simplified PMSM Drive/LConn2
  C/RConn1 -- Simplified PMSM Drive/RConn3

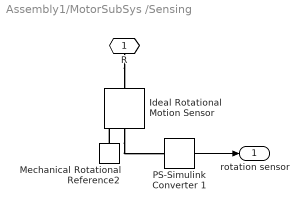
== system Assembly1/MotorSubSys /Sensing ==
  Ideal Rotational Motion Sensor : fl_lib/Mechanical/Mechanical Sensors/Ideal Rotational Motion Sensor  offset=0 rad
  Mechanical Rotational Reference2 : fl_lib/Mechanical/Rotational Elements/Mechanical Rotational Reference
  PS-Simulink Converter 1 : nesl_utility/PS-Simulink Converter  PhysicalDomain=network_engine_domain  SubClassName=ps_output  LeftPortType=input  RightPortType=output  PseudoPeriodic=off  Frequencies=[]  Unit=rpm  AffineConversion=off
  R : PMIOPort  Side=Left
  "rotation sensor " : Outport  VectorParamsAs1DForOutWhenUnconnected=off
  wires:
  PS-Simulink Converter 1/1 -> "rotation sensor "/1
  connections:
  Ideal Rotational Motion Sensor/RConn2 -- PS-Simulink Converter 1/LConn1
  Mechanical Rotational Reference2/LConn1 -- Ideal Rotational Motion Sensor/RConn1
  R/RConn1 -- Ideal Rotational Motion Sensor/LConn1

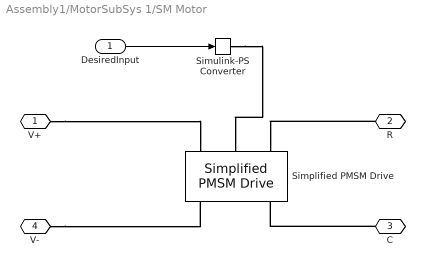
== system Assembly1/MotorSubSys 1/SM Motor ==
  "DesiredInput " : Inport
  Simplified PMSM Drive : ee_lib/Electromechanical/Permanent Magnet/Simplified PMSM Drive  torque_speed_param=2  w_t=[0, 3750, 7500, 8000] rpm  T_t=[.09, .08, .07, 0] N*m  torque_max=1490 mN*m  power_max=285.6 W  Tc=7.99 ms  losses_param=1  eff=86.5  w_eff=1960 rpm  T_eff=65.373 mN*m  Piron=1.8338 W  Pbase=0 W  w_eff_vec=[-8000, -4000, 0, 4000, 8000] rpm  T_eff_vec=[0, .03, .06, .09] N*m  v_eff_vec=[100, 250, 400] V  losses_mat=[1.49, 1.67, 2.21, 3.1; .42, .69, 1.14, 2.03; .06, .24, .78, 1.68; .42, .69, 1.14, 2.03; 1.49, 1.67, 2.21, 3.1] W  efficiency_mat=[95, 95, 95, 95; 95, 95, 95, 95; 95, 95, 95, 95; 95, 95, 95, 95; 95, 95, 95, 95]  losses_mat_3D=ones(5, 4, 3) W  efficiency_mat_3D=95 * ones(5, 4, 3)  Res=0 Ohm  J=5100 g*cm^2  lam=1e-5 N*m/(rad/s)  speed0=0 rpm  faulted_specify=off  faulted_priority=None  faulted=0  faulted_nominal_specify=off  faulted_nominal_unit=1  faulted_nominal_value=1  alpha=3.93e-3 1/K  Tmeas=25 degC  Tmeas2=125 degC  losses_mat_T2=[1.49, 1.74, 2.49, 3.74; .42, .67, 1.42, 2.67; .06, .31, 1.06, 2.31; .42, .67, 1.42, 2.67; 1.49, 1.74, 2.49, 3.74] W  efficiency_mat_T2=[95, 95, 95, 95; 95, 95, 95, 95; 95, 95, 95, 95; 95, 95, 95, 95; 95, 95, 95, 95]  losses_mat_3D_T2=ones(5, 4, 3) W  efficiency_mat_3D_T2=95 * ones(5, 4, 3)  thermal_mass=100 J/K  initial_temperature=25 degC  fault_condition=1  fault_threshold=0.5
      settings: SourceProductName=Simscape Electrical  SourceProductBaseCode=PS  InternalSimscapePortConfiguration="{\"Bottom\":[],\"Left\":[{\"id\":\"Vp\",\"label\":\"+\",\"type\":\"foundation.electrical.electrical\"},{\"id\":\"Tr\",\"label\":\"Tr\",\"type\":\"input\"},{\"id\":\"R\",\"label\":\"R\",\"type\":\"foundation.mechanical.rotational.rotational\"}],\"Right\":[{\"id\":\"Vm\",\"label\":\"-\",\"type\":\"foundation.electrical.electrical\"},{\"id\":\"Omega\",\"label\":\"w\",\"type\":\"output\"},{\"id\":\"C\",\"label\":\"C\",\"type\":\"foundation.mechanical.rotational.rotational\"}],\"Top\":[]}"
  Simulink-PS Converter : nesl_utility/Simulink-PS Converter  PhysicalDomain=network_engine_domain  SubClassName=ps_input  LeftPortType=input  RightPortType=output  PseudoPeriodic=off  Frequencies=[]  NoiseDistribution=none  NoiseParameters=[]  Unit=1  AffineConversion=off  FilteringAndDerivatives=provide  SimscapeFilterOrder=1  InputFilterTimeConstant=0.001  UdotUserProvided=0
  V+ : PMIOPort  Side=Left
  R : PMIOPort  Port=2  Side=Right
  C : PMIOPort  Port=3  Side=Right
  V- : PMIOPort  Port=4  Side=Left
  wires:
  "DesiredInput "/1 -> Simulink-PS Converter/1
  connections:
  V-/RConn1 -- Simplified PMSM Drive/RConn1
  V+/RConn1 -- Simplified PMSM Drive/LConn1
  R/RConn1 -- Simplified PMSM Drive/LConn3
  Simulink-PS Converter/RConn1 -- Simplified PMSM Drive/LConn2
  C/RConn1 -- Simplified PMSM Drive/RConn3

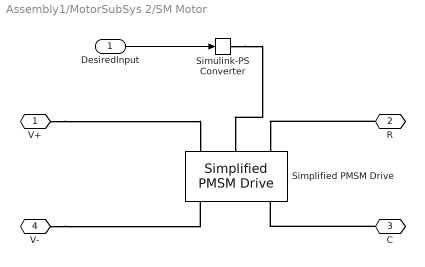
== system Assembly1/MotorSubSys 2/SM Motor ==
  "DesiredInput " : Inport
  Simplified PMSM Drive : ee_lib/Electromechanical/Permanent Magnet/Simplified PMSM Drive  torque_speed_param=2  w_t=[0, 3750, 7500, 8000] rpm  T_t=[.09, .08, .07, 0] N*m  torque_max=1490 mN*m  power_max=285.6 W  Tc=7.99 ms  losses_param=1  eff=86.5  w_eff=1960 rpm  T_eff=65.373 mN*m  Piron=1.8338 W  Pbase=0 W  w_eff_vec=[-8000, -4000, 0, 4000, 8000] rpm  T_eff_vec=[0, .03, .06, .09] N*m  v_eff_vec=[100, 250, 400] V  losses_mat=[1.49, 1.67, 2.21, 3.1; .42, .69, 1.14, 2.03; .06, .24, .78, 1.68; .42, .69, 1.14, 2.03; 1.49, 1.67, 2.21, 3.1] W  efficiency_mat=[95, 95, 95, 95; 95, 95, 95, 95; 95, 95, 95, 95; 95, 95, 95, 95; 95, 95, 95, 95]  losses_mat_3D=ones(5, 4, 3) W  efficiency_mat_3D=95 * ones(5, 4, 3)  Res=0 Ohm  J=5100 g*cm^2  lam=1e-5 N*m/(rad/s)  speed0=0 rpm  faulted_specify=off  faulted_priority=None  faulted=0  faulted_nominal_specify=off  faulted_nominal_unit=1  faulted_nominal_value=1  alpha=3.93e-3 1/K  Tmeas=25 degC  Tmeas2=125 degC  losses_mat_T2=[1.49, 1.74, 2.49, 3.74; .42, .67, 1.42, 2.67; .06, .31, 1.06, 2.31; .42, .67, 1.42, 2.67; 1.49, 1.74, 2.49, 3.74] W  efficiency_mat_T2=[95, 95, 95, 95; 95, 95, 95, 95; 95, 95, 95, 95; 95, 95, 95, 95; 95, 95, 95, 95]  losses_mat_3D_T2=ones(5, 4, 3) W  efficiency_mat_3D_T2=95 * ones(5, 4, 3)  thermal_mass=100 J/K  initial_temperature=25 degC  fault_condition=1  fault_threshold=0.5
      settings: SourceProductName=Simscape Electrical  SourceProductBaseCode=PS  InternalSimscapePortConfiguration="{\"Bottom\":[],\"Left\":[{\"id\":\"Vp\",\"label\":\"+\",\"type\":\"foundation.electrical.electrical\"},{\"id\":\"Tr\",\"label\":\"Tr\",\"type\":\"input\"},{\"id\":\"R\",\"label\":\"R\",\"type\":\"foundation.mechanical.rotational.rotational\"}],\"Right\":[{\"id\":\"Vm\",\"label\":\"-\",\"type\":\"foundation.electrical.electrical\"},{\"id\":\"Omega\",\"label\":\"w\",\"type\":\"output\"},{\"id\":\"C\",\"label\":\"C\",\"type\":\"foundation.mechanical.rotational.rotational\"}],\"Top\":[]}"
  Simulink-PS Converter : nesl_utility/Simulink-PS Converter  PhysicalDomain=network_engine_domain  SubClassName=ps_input  LeftPortType=input  RightPortType=output  PseudoPeriodic=off  Frequencies=[]  NoiseDistribution=none  NoiseParameters=[]  Unit=1  AffineConversion=off  FilteringAndDerivatives=provide  SimscapeFilterOrder=1  InputFilterTimeConstant=0.001  UdotUserProvided=0
  V+ : PMIOPort  Side=Left
  R : PMIOPort  Port=2  Side=Right
  C : PMIOPort  Port=3  Side=Right
  V- : PMIOPort  Port=4  Side=Left
  wires:
  "DesiredInput "/1 -> Simulink-PS Converter/1
  connections:
  V-/RConn1 -- Simplified PMSM Drive/RConn1
  V+/RConn1 -- Simplified PMSM Drive/LConn1
  R/RConn1 -- Simplified PMSM Drive/LConn3
  Simulink-PS Converter/RConn1 -- Simplified PMSM Drive/LConn2
  C/RConn1 -- Simplified PMSM Drive/RConn3

== matlab function Assembly1/MATLAB Function1 ==
  data: var1 input; outputArray output; var2 input; var3 input
function outputArray = collate(var1, var2, var3)

outputArray = [var1,var2,var3];

== matlab function Assembly1/MATLAB Function ==
  data: xPos output; yPos output; dimensions input; angles input; ctrl_1 output; Dd input; Kd input; xd input; xd_dot input; ctrl_2 output; ctrl_3 output; xd_ddot input; stiffnessBit output; dampingBit output; inertiaBit output
function [xPos, yPos, ctrl_1, ctrl_2, ctrl_3, stiffnessBit, dampingBit, inertiaBit] = LinkSimpleImpedanceCtrl(dimensions, angles, Dd, Kd, xd, xd_dot, xd_ddot)

ang1 = angles(1);
ang2 = angles(2);
ang3 = angles(3);
L1 = dimensions(1);
L2 = dimensions(2);
L3 = dimensions(3);


xPos = (L1*cos(ang1) + L2*cos(ang1 + ang2) + L3*cos(ang1 + ang2 + ang3));
yPos = (L1*sin(ang1) + L2*sin(ang1 + ang2) + L3*sin(ang1 + ang2 + ang3));

%diff of x and y formulae
x_dot = double(- L2*sin(ang1 + ang2) - L1*sin(ang1) - L3*sin(ang1 + ang2 + ang3));
y_dot = double(L2*cos(ang1 + ang2) + L1*cos(ang1) + L3*cos(ang1 + ang2 + ang3));

x_ddot = double(- L2*cos(ang1 + ang2) - L1*cos(ang1) - L3*cos(ang1 + ang2 + ang3));
y_ddot = double(- L2*sin(ang1 + ang2) - L1*sin(ang1) - L3*sin(ang1 + ang2 + ang3));

%Calculated J and then the transpose 
J_T = [ - L2*sin(ang1 + ang2) - L1*sin(ang1) - L3*sin(ang1 + ang2 + ang3), L2*cos(ang1 + ang2) + L1*cos(ang1) + L3*cos(ang1 + ang2 + ang3), 0;
                - L2*sin(ang1 + ang2) - L3*sin(ang1 + ang2 +ang3),                L2*cos(ang1 + ang2) + L3*cos(ang1 + ang2 + ang3), 0;
                                      -L3*sin(ang1 + ang2 + ang3),                                      L3*cos(ang1 + ang2 + ang3), 0];


pos = [xPos; yPos; 0] ;
pos_dot = [x_dot; y_dot; 0];
pos_ddot = [x_ddot; y_ddot; 0];


Im = [ (L2*cos(ang1 + ang2) + L1*cos(ang1))*((4322095789375391*cos(conj(ang1))*conj(L1))/18014398509481984 + (4322095789375391*cos(conj(ang1) + conj(ang2))*conj(L2))/18014398509481984) + (L2*sin(ang1 + ang2) + L1*sin(ang1) + L3*sin(ang1 + ang2 + ang3))*((5653631132464783*sin(conj(ang1) + conj(ang2) + conj(ang3))*conj(L3))/72057594037927936 + (5653631132464783*sin(conj(ang1))*conj(L1))/72057594037927936 + (5653631132464783*sin(conj(ang1) + conj(ang2))*conj(L2))/72057594037927936) + (L2*sin(ang1 + ang2) + L1*sin(ang1))*((4322095789375391*sin(conj(ang1))*conj(L1))/18014398509481984 + (4322095789375391*sin(conj(ang1) + conj(ang2))*conj(L2))/18014398509481984) + (L2*cos(ang1 + ang2) + L1*cos(ang1) + L3*cos(ang1 + ang2 + ang3))*((5653631132464783*cos(conj(ang1) + conj(ang2) + conj(ang3))*conj(L3))/72057594037927936 + (5653631132464783*cos(conj(ang1))*conj(L1))/72057594037927936 + (5653631132464783*cos(conj(ang1) + conj(ang2))*conj(L2))/72057594037927936) + (4516478355052105*L1*cos(conj(ang1))*conj(L1)*cos(ang1))/18014398509481984 + (4516478355052105*L1*sin(conj(ang1))*conj(L1)*sin(ang1))/18014398509481984, (L2*cos(ang1 + ang2) + L3*cos(ang1 + ang2 + ang3))*((5653631132464783*cos(conj(ang1) + conj(ang2) + conj(ang3))*conj(L3))/72057594037927936 + (5653631132464783*cos(conj(ang1))*conj(L1))/72057594037927936 + (5653631132464783*cos(conj(ang1) + conj(ang2))*conj(L2))/72057594037927936) + (L2*sin(ang1 + ang2) + L3*sin(ang1 + ang2 + ang3))*((5653631132464783*sin(conj(ang1) + conj(ang2) + conj(ang3))*conj(L3))/72057594037927936 + (5653631132464783*sin(conj(ang1))*conj(L1))/72057594037927936 + (5653631132464783*sin(conj(ang1) + conj(ang2))*conj(L2))/72057594037927936) + L2*sin(ang1 + ang2)*((4322095789375391*sin(conj(ang1))*conj(L1))/18014398509481984 + (4322095789375391*sin(conj(ang1) + conj(ang2))*conj(L2))/18014398509481984) + L2*cos(ang1 + ang2)*((4322095789375391*cos(conj(ang1))*conj(L1))/18014398509481984 + (4322095789375391*cos(conj(ang1) + conj(ang2))*conj(L2))/18014398509481984), L3*cos(ang1 + ang2 + ang3)*((5653631132464783*cos(conj(ang1) + conj(ang2) + conj(ang3))*conj(L3))/72057594037927936 + (5653631132464783*cos(conj(ang1))*conj(L1))/72057594037927936 + (5653631132464783*cos(conj(ang1) + conj(ang2))*conj(L2))/72057594037927936) + L3*sin(ang1 + ang2 + ang3)*((5653631132464783*sin(conj(ang1) + conj(ang2) + conj(ang3))*conj(L3))/72057594037927936 + (5653631132464783*sin(conj(ang1))*conj(L1))/72057594037927936 + (5653631132464783*sin(conj(ang1) + conj(ang2))*conj(L2))/72057594037927936);
    ((5653631132464783*sin(conj(ang1) + conj(ang2) + conj(ang3))*conj(L3))/72057594037927936 + (5653631132464783*sin(conj(ang1) + conj(ang2))*conj(L2))/72057594037927936)*(L2*sin(ang1 + ang2) + L1*sin(ang1) + L3*sin(ang1 + ang2 + ang3)) + ((5653631132464783*cos(conj(ang1) + conj(ang2) + conj(ang3))*conj(L3))/72057594037927936 + (5653631132464783*cos(conj(ang1) + conj(ang2))*conj(L2))/72057594037927936)*(L2*cos(ang1 + ang2) + L1*cos(ang1) + L3*cos(ang1 + ang2 + ang3)) + (4322095789375391*cos(conj(ang1) + conj(ang2))*conj(L2)*(L2*cos(ang1 + ang2) + L1*cos(ang1)))/18014398509481984 + (4322095789375391*sin(conj(ang1) + conj(ang2))*conj(L2)*(L2*sin(ang1 + ang2) + L1*sin(ang1)))/18014398509481984,                                                                                                                                                                                                                                                                     ((5653631132464783*cos(conj(ang1) + conj(ang2) + conj(ang3))*conj(L3))/72057594037927936 + (5653631132464783*cos(conj(ang1) + conj(ang2))*conj(L2))/72057594037927936)*(L2*cos(ang1 + ang2) + L3*cos(ang1 + ang2 + ang3)) + ((5653631132464783*sin(conj(ang1) + conj(ang2) + conj(ang3))*conj(L3))/72057594037927936 + (5653631132464783*sin(conj(ang1) + conj(ang2))*conj(L2))/72057594037927936)*(L2*sin(ang1 + ang2) + L3*sin(ang1 + ang2 + ang3)) + (4322095789375391*L2*cos(conj(ang1) + conj(ang2))*cos(ang1 + ang2)*conj(L2))/18014398509481984 + (4322095789375391*L2*sin(conj(ang1) + conj(ang2))*sin(ang1 + ang2)*conj(L2))/18014398509481984,                                                                                                                                 L3*cos(ang1 + ang2 + ang3)*((5653631132464783*cos(conj(ang1) + conj(ang2) + conj(ang3))*conj(L3))/72057594037927936 + (5653631132464783*cos(conj(ang1) + conj(ang2))*conj(L2))/72057594037927936) + L3*sin(ang1 + ang2 + ang3)*((5653631132464783*sin(conj(ang1) + conj(ang2) + conj(ang3))*conj(L3))/72057594037927936 + (5653631132464783*sin(conj(ang1) + conj(ang2))*conj(L2))/72057594037927936);
    (5653631132464783*cos(conj(ang1) + conj(ang2) + conj(ang3))*conj(L3)*(L2*cos(ang1 + ang2) + L1*cos(ang1) + L3*cos(ang1 + ang2 + ang3)))/72057594037927936 + (5653631132464783*sin(conj(ang1) + conj(ang2) + conj(ang3))*conj(L3)*(L2*sin(ang1 + ang2) + L1*sin(ang1) + L3*sin(ang1 + ang2 + ang3)))/72057594037927936,                                                                                                                                                                                                                                                                                                                                                                                                                                                                                                                                                                                                                                     (5653631132464783*cos(conj(ang1) + conj(ang2) + conj(ang3))*conj(L3)*(L2*cos(ang1 + ang2) + L3*cos(ang1 + ang2 + ang3)))/72057594037927936 + (5653631132464783*sin(conj(ang1) + conj(ang2) + conj(ang3))*conj(L3)*(L2*sin(ang1 + ang2) + L3*sin(ang1 + ang2 + ang3)))/72057594037927936,                                                                                                                                                                                                                                                          (5653631132464783*L3*cos(conj(ang1) + conj(ang2) + conj(ang3))*conj(L3)*cos(ang1 + ang2 + ang3))/72057594037927936 + (5653631132464783*L3*sin(conj(ang1) + conj(ang2) + conj(ang3))*conj(L3)*sin(ang1 + ang2 + ang3))/72057594037927936 + 970850075628535821/549755813888000];
 


%controlTorque = subs(J_T) * (Kd(xd - pos) + Dd(xd_dot - pos_dot));
stiffnessBit = Kd * (xd - pos);
dampingBit = Dd*(xd_dot - pos_dot);
inertiaBit = Im*(xd_ddot - pos_ddot);
controlTorques =  J_T*(inertiaBit + stiffnessBit + dampingBit);

ctrl_1 = controlTorques(1);
ctrl_2 = double(controlTorques(2));
ctrl_3 = double(controlTorques(3));

== matlab function Assembly1/MATLAB Function2 ==
  data: var1 input; outputArray output; var2 input; var3 input
function outputArray = collate(var1, var2, var3)

outputArray = [var1,var2,var3];
